simulink model "ds_capital_linear_1o_simulation_notint_simu"  (R2022b)
settings: Solver=FixedStepAuto  StartTime=0.0  StopTime=N*time_step  FixedStep=5  RelTol=1e-3
values from neighbouring files (symbols this model uses):
  A = temp.A    [ds_capital_linear_1o_simulation_notint.m]    (also in ds_capital_linear_1o_simulation_notint_data.mat = 1)
  B = temp.B    [ds_capital_linear_1o_simulation_notint.m]    (also in ds_capital_linear_1o_simulation_notint_data.mat = [0.0272685899265 0.0272685899265 0.0272685899265 -0.02726858)
  C = temp.C    [ds_capital_linear_1o_simulation_notint.m]    (also in ds_capital_linear_1o_simulation_notint_data.mat = 0.125)
  D = temp.D    [ds_capital_linear_1o_simulation_notint.m]    (also in ds_capital_linear_1o_simulation_notint_data.mat = [0.00121707459429 0.00360643085568 0.0116055992339 -0.182051)
  K_constant = 0.721578991791    [ds_capital_linear_1o_simulation_notint_data.mat]
  Q0or = 0.513349020699    [ds_capital_linear_1o_simulation_notint_data.mat]
  YX = 0.853229730498    [ds_capital_linear_1o_simulation_notint_data.mat]
settings Model: Creator=chuan  LastModifiedBy=chuan

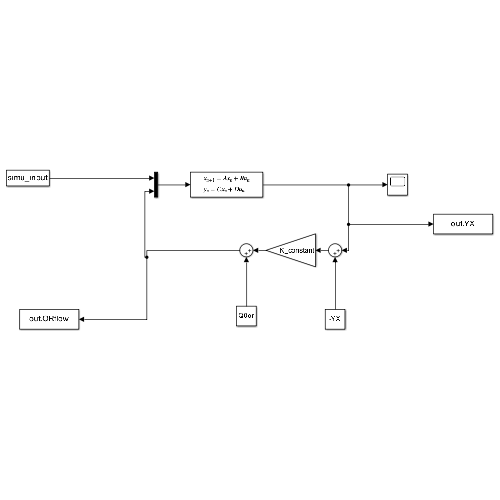
[thumbnail: Simulink's stored preview of the top-level diagram]
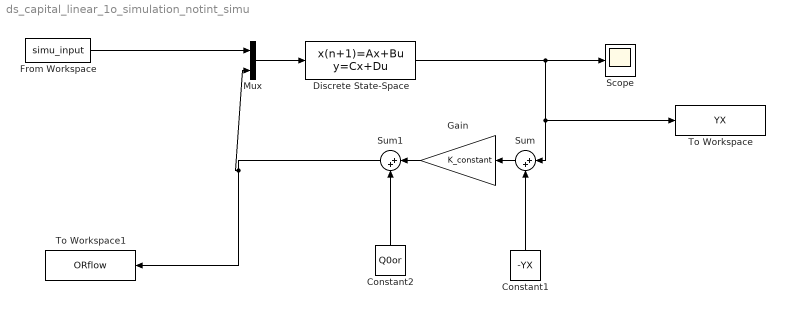
== system ds_capital_linear_1o_simulation_notint_simu ==
  Constant1 : Constant  Value=-YX
  Constant2 : Constant  Value=Q0or
  Discrete State-Space : DiscreteStateSpace  A=A  B=B  C=C  D=D  SampleTime=-1
  From Workspace : FromWorkspace  VariableName=simu_input  SampleTime=-1
  Gain : Gain  Gain=K_constant
  Mux : Mux  Inputs=2
  Scope : Scope
  Sum : Sum  Inputs=|++
  Sum1 : Sum  Inputs=|++
  To Workspace : ToWorkspace  VariableName=YX  SaveFormat=Timeseries  SampleTime=-1
  To Workspace1 : ToWorkspace  VariableName=ORflow  SaveFormat=Timeseries  SampleTime=-1
  wires:
  Discrete State-Space/1 -> Sum/1, To Workspace/1, Scope/1
  Mux/1 -> Discrete State-Space/1
  From Workspace/1 -> Mux/1
  Constant1/1 -> Sum/2
  Constant2/1 -> Sum1/2
  Gain/1 -> Sum1/1
  Sum/1 -> Gain/1
  Sum1/1 -> To Workspace1/1, Mux/2
